simulink model "DriverPath"  (R2025a)
settings: Solver=ode4  StartTime=0.0  StopTime=120  FixedStep=2e-4  RelTol=1e-3
model workspace (MAT data in the model file):
  drvDelayGain = 0.2
  drvKff = 0
  drvKi = 2
  drvKp = 8
  drvN = 4586
  drvNlim = 4
  drvPlanAyCap = 8.6
  drvPlanBrkMargin = 0.6
  drvPlanFW = [-25 -25 -25 -25 -25 -25 -25 -25 -25 -25 -25 -25 ... (4586 elements, 4586x1)]
  drvPlanFzOffN = 0
  drvPlanRH = [10 15 20 25 30 35 40 45 50 55 65 80 ... (39 elements, 13x3)]
  drvPlanRW = [-10 -10 -10 -10 -10 -10 -10 -10 -10 -10 -10 -10 ... (4586 elements, 4586x1)]
  drvPosGainF = 2.5
  drvPosGainR = 2.5
  drvPreviewL = 10
  drvRefKap = [7.37152757629e-05 7.69388209234e-05 7.92839882257e-05 8.08057927362e-05 8.16087590431e-05 8.200862796e-05 8.24299237596e-05 5.11331855999e-05 -0.000149124545088 -0.000317829936074 -0.000343270987749 -0.00029252411928 ... (4586 elements, 4586x1)]
  drvRefPsi = [0 -0.00101392427346 -0.00488065271301 -0.00770746494827 -0.00765908209454 -0.00761399605665 -0.00756111206845 -0.0074887410786 -0.00740766580275 -0.00731954306241 -0.00722036808131 -0.0071279710415 ... (4586 elements, 4586x1)]
  drvRefVplan = [72.4966611223 72.633405974 72.7695456132 72.9050859541 73.0400328206 73.1743919474 73.3081689827 73.4413694893 73.5739989467 73.706062753 73.8375662259 73.968514605 ... (4586 elements, 4586x1)]
  drvRefVraw = [82.8119463936 82.9460939647 83.1011358314 83.2592394893 83.4173431472 83.5753892782 83.7129621785 83.850455756 83.9879220862 84.1191136363 84.2060523792 84.2966104987 ... (4586 elements, 4586x1)]
  drvRefX = [0 0.999999998224 1.99999171552 2.99996181238 3.99993230962 4.99990315023 5.99987433602 6.99984597813 7.99981825196 8.99979110191 9.9997646721 10.999738964 ... (4586 elements, 4586x1)]
  drvRefY = [0 0 -0.00202784084198 -0.0097611965607 -0.0174426181092 -0.0250792109788 -0.0326704630805 -0.0402012910107 -0.0476478052224 -0.0550164870998 -0.0622867605989 -0.0694570977558 ... (4586 elements, 4586x1)]
  drvSFa = 0.9
  drvSFb = 0.9
  drvSpeedLook = 15
  drvTau = 0.05
  drvUsePlan = 1
  drvVScale = 0.95
  drvVnom = 60
  drvVx0 = 82.8119463936
  drvYawGain = 0.2
undefined symbols (not defined in the file): driverTyreGrip, pt, vp
libraries: vehdynlibdriver x1
(part 2 of 2)

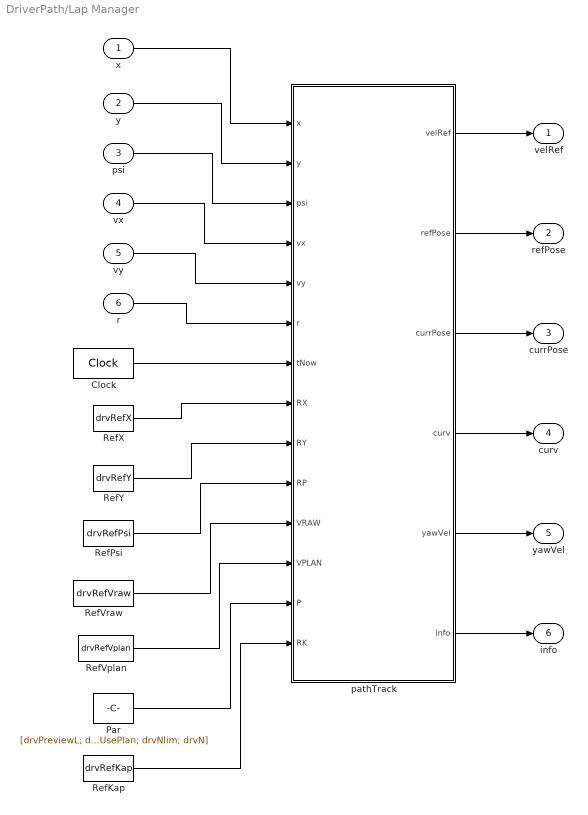
== system DriverPath/Lap Manager ==
  x : Inport
  y : Inport  Port=2
  psi : Inport  Port=3
  vx : Inport  Port=4
  vy : Inport  Port=5
  r : Inport  Port=6
  Clock : DigitalClock  Description=Simulation time, for the lap timer.  SampleTime=0.001
  Par : Constant  Description=Lap Manager parameter vector: [previewL; speedLook; vScale; usePlan; nLim; N]. The last element is the reference-array length drvN -- it was a LITERAL 4586 (Barcelona) until 2026-09-21, which pinned the whole model to one track. drvN is written with drvRefX/Y/Psi/Kap/Vraw/Vplan by simulink/tools/applyTrackPack.m.  Value=[drvPreviewL; drvSpeedLook; drvVScale; drvUsePlan; drvNlim; drvN]
  RefKap : Constant  Description=Racing-line curvature [1/m], ISO sign (+ = LEFT turn), chord-estimated over +-10 m. Feeds the Stanley controller's Curvature port (negated to SAE).  Value=drvRefKap
  RefPsi : Constant  Description=Racing line heading [rad], unwrapped.  Value=drvRefPsi
  RefVplan : Constant  Description=|  Value=drvRefVplan
      | Grip- and feasibility-limited speed profile [m/s]. Built by
      | simulink/tools/buildSpeedPlan.m from the live MF5.2 tyre law, the live
      | ride-height aero and the ECU's own wing-station law; regenerate it with
      | simulink/tools/rebuildDriverPlan.m, which is the supported route and the only
      | TRACKED one (simulink/work/ is git-ignored).
      | 
      | PROVENANCE -- every input is stored beside this vector in the model workspace,
      | and rebuildDriverPlan.m reads AND writes each one, so the plan is exactly
      | reproducible on a fresh clone:
      |   drvPlanRH        measured ride-height-vs-speed table [v RHf RHr]. Must span
      |                    the speeds the car actually reaches -- a table that stops
      |                    short is held at its top row, and held short it once
      |                    predicted ClF = +0.10 at 85-90 m/s where the plant measures
      |                    +0.42, i.e. four times the front LIFT, in the fastest part
      |                    of the lap.
      |   drvPlanAyCap     DRIVER-MODEL lateral ceiling [m/s^2]. The single largest
      |                    lap-time term. It is a limitation of the forward-time
      |                    Stanley + pedal-map driver, NOT a vehicle or aerodynamic
      |                    limit, and must never be quoted as one; raise it when the
      |                    lateral controller improves.
      |   drvPlanFzOffN    residual constant front-axle load transfer [N], ADDITIVE on
      |                    the static load only (never a multiplicative derate of
      |                    static+aero, which would discount front downforce).
      |   drvPlanBrkMargin decel-budget fraction [-].
      |   drvPlanRW/FW     the wing station the ECU's law commands at each point,
      |                    recorded so the plan's aerodynamic assumption is auditable.
      | 
      | The former drvPlanFzF (a multiplicative front derate) is DELETED -- it scaled
      | aerodynamic front load down along with the static load, understating exactly
      | the quantity this project measures.
  RefVraw : Constant  Description=ref.vx(s), the solved ARFWr speed profile [m/s], untouched.  Value=drvRefVraw
  RefX : Constant  Description=Racing line X [m], 1 m uniform, plant start frame.  Value=drvRefX
  RefY : Constant  Description=Racing line Y [m].  Value=drvRefY
  pathTrack : MATLAB Function  TreatAsAtomicUnit=on
  velRef : Outport
  refPose : Outport  Port=2
  currPose : Outport  Port=3
  curv : Outport  Port=4
  yawVel : Outport  Port=5
  info : Outport  Port=6
  wires:
  x/1 -> pathTrack/1(x)
  r/1 -> pathTrack/6(r)
  psi/1 -> pathTrack/3(psi)
  RefVplan/1 -> pathTrack/12(VPLAN)
  y/1 -> pathTrack/2(y)
  vy/1 -> pathTrack/5(vy)
  vx/1 -> pathTrack/4(vx)
  RefX/1 -> pathTrack/8(RX)
  Clock/1 -> pathTrack/7(tNow)
  RefY/1 -> pathTrack/9(RY)
  RefPsi/1 -> pathTrack/10(RP)
  RefVraw/1 -> pathTrack/11(VRAW)
  Par/1 -> pathTrack/13(P)
  RefKap/1 -> pathTrack/14(RK)
  pathTrack/1(velRef) -> velRef/1
  pathTrack/2(refPose) -> refPose/1
  pathTrack/4(curv) -> curv/1
  pathTrack/3(currPose) -> currPose/1
  pathTrack/5(yawVel) -> yawVel/1
  pathTrack/6(info) -> info/1

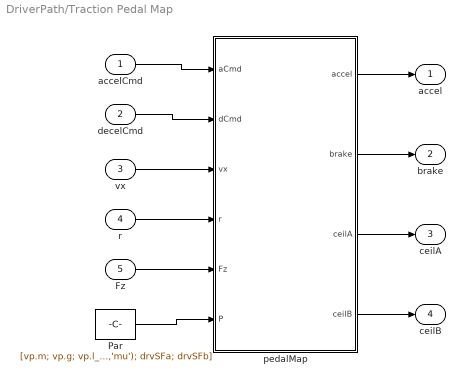
== system DriverPath/Traction Pedal Map ==
  accelCmd : Inport
  decelCmd : Inport  Port=2
  vx : Inport  Port=3
  r : Inport  Port=4
  Fz : Inport  Port=5
  Par : Constant  Description=|  Value=[vp.m; vp.g; vp.l_f; vp.l_r; vp.l; vp.Rw; vp.Tdist; pt.Tmax; vp.gear; pt.Pmax; 1; vp.Tbrake_max; vp.brkB; driverTyreGrip(vp,'mu'); drvSFa; drvSFb]
      | Traction pedal-map parameters, IN THIS ORDER (pedalMap reads them by index):
      |  1 vp.m           mass [kg]
      |  2 vp.g           gravity [m/s^2]
      |  3 vp.l_f         CG -> front axle [m]
      |  4 vp.l_r         CG -> rear axle [m]
      |  5 vp.l           wheelbase [m]
      |  6 vp.Rw          wheel radius [m]
      |  7 vp.Tdist       REAR torque fraction [-]      Parameters/vehParams.m:20
      |  8 pt.Tmax        machine torque cap [Nm]       Parameters/Powertrain.m:80
      |  9 vp.gear        single ratio [-]              Parameters/Powertrain.m:67
      | 10 pt.Pmax        wheel-side power cap [W]      Parameters/Powertrain.m:53
      | 11 Om floor       [rad/s], guards Pmax/Om at standstill -- a numerical guard,
      |                   the one literal in this vector (same role as torqueStep's)
      | 12 vp.Tbrake_max  brake channel cap [Nm]        Parameters/vehParams.m:344
      | 13 vp.brkB        FRONT brake fraction [-]      Parameters/vehParams.m:19
      | 14 muX            PLACEHOLDER tyre peak long. friction (build-time read-back)
      | 15 muY            PLACEHOLDER tyre peak lat. friction  (build-time read-back)
      | 16 drvSFa         accel safety factor [-]  TUNABLE
      | 17 drvSFb         brake safety factor [-]  TUNABLE
  pedalMap : MATLAB Function  TreatAsAtomicUnit=on
  accel : Outport
  brake : Outport  Port=2
  ceilA : Outport  Port=3
  ceilB : Outport  Port=4
  wires:
  accelCmd/1 -> pedalMap/1(aCmd)
  Fz/1 -> pedalMap/5(Fz)
  r/1 -> pedalMap/4(r)
  vx/1 -> pedalMap/3(vx)
  decelCmd/1 -> pedalMap/2(dCmd)
  Par/1 -> pedalMap/6(P)
  pedalMap/1(accel) -> accel/1
  pedalMap/2(brake) -> brake/1
  pedalMap/3(ceilA) -> ceilA/1
  pedalMap/4(ceilB) -> ceilB/1

== matlab function DriverPath/Traction Pedal Map/pedalMap ==
  data: aCmd input; accel output; dCmd input; vx input; r input; Fz input; P input; brake output; ceilA output; ceilB output
function [accel, brake, ceilA, ceilB] = pedalMap(aCmd, dCmd, vx, r, Fz, P)
%#codegen
% Friction-ellipse pedal map. See the subsystem description for the full
% derivation and for WHY this is a multiplicative map and not a clamp.
%
% P = [m; g; l_f; l_r; l; Rw; Tdist; Tmax; gear; Pmax; OmFloor; Tbmax; brkB;
%      muX; muY; SFa; SFb]

mm  = P(1);  lf = P(3);  lr = P(4);  ll = P(5);  Rw = P(6);
Tds = P(7);  Tmx = P(8); gr = P(9);  Pmx = P(10); OmFl = P(11);
Tbm = P(12); brk = P(13); muX = P(14); muY = P(15); SFa = P(16); SFb = P(17);

Fzf = Fz(1) + Fz(2);
Fzr = Fz(3) + Fz(4);

% lateral demand: steady-state ay = vx*r. vx and r are body-integrator
% outputs, so this closes no algebraic loop (VehStateBus.ay would).
ay  = vx*r;
FyF = mm*ay*lr/ll;
FyR = mm*ay*lf/ll;
kxy = muX/muY;

capF = sqrt(max((muX*Fzf)^2 - (kxy*FyF)^2, 0));
capR = sqrt(max((muX*Fzr)^2 - (kxy*FyR)^2, 0));

% drive: same envelope Plant/Torque Path/torqueStep applies
OmM   = max(vx/Rw, OmFl);
TwCap = min(Tmx*gr, Pmx/OmM);
dmdAF = TwCap*(1 - Tds)/Rw;
dmdAR = TwCap*Tds/Rw;
ceilA = min([SFa*capF/max(dmdAF, 1), SFa*capR/max(dmdAR, 1), 1]);

% brake: torqueStep applies T_brake*brkB per FRONT wheel (two wheels)
dmdBF = 2*Tbm*brk/Rw;
dmdBR = 2*Tbm*(1 - brk)/Rw;
ceilB = min([SFb*capF/max(dmdBF, 1), SFb*capR/max(dmdBR, 1), 1]);

ceilA = max(ceilA, 0);
ceilB = max(ceilB, 0);

accel = min(max(aCmd, 0), 1)*ceilA;
brake = min(max(dCmd, 0), 1)*ceilB;

== matlab function DriverPath/Lap Manager/pathTrack ==
  data: x input; velRef output; y input; psi input; vx input; vy input; r input; tNow input; RX input; RY input; RP input; VRAW input; VPLAN input; P input; RK input; refPose output; currPose output; curv output; yawVel output; info output
function [velRef, refPose, currPose, curv, yawVel, info] = pathTrack( ...
        x, y, psi, vx, vy, r, tNow, RX, RY, RP, VRAW, VPLAN, P, RK)
%#codegen
% Path tracker + lap manager.
%
% FRAME: the plant bus, the stored reference and every quantity on LapInfo are
% ISO 8855 (x fwd, y LEFT, psi/r CCW +). The VDB Predictive Driver's Stanley
% controller uses SAE J670 (Z-down): its pose angle is CLOCKWISE positive and
% its hidden coordMode is fixed at "SAE J670 (Z-down)". So the four signals
% handed to the block -- refPose, currPose, curv, yawVel -- are MIRRORED here
% (y, psi, kappa, r all negate; x does not), and the block's SteerCmd is
% mirrored back by the NEGATIVE gain in the Steer scale block. This is the only
% place the driver-side mirror happens, exactly as Plant's Vehicle State Bus
% subsystem is the only place the plant-side mirror happens.
%
% The reference grid is EXACTLY 1 m, closed, so arc length == index - 1.
%
% P = [previewL; speedLook; vScale; usePlan; nLim; N]

Lp   = P(1);  Lv = P(2);  vSc = P(3);  usePlan = P(4);  nLim = P(5);
N    = int32(P(6));

persistent iPrev tStart lapCnt lastLap maxN acquired
if isempty(acquired)
    iPrev = int32(1); tStart = 0; lapCnt = 0; lastLap = 0; maxN = 0;
    acquired = false;
end

% ---- nearest reference point -----------------------------------------
% First step: full search (the car may be started anywhere). After that a
% short forward window is enough -- ds is 1 m and the car covers at most
% 0.12 m per 1 ms step at the reference's peak speed.
best = int32(1); bestD = realmax;
if ~acquired
    for k = 1:N
        dxk = RX(k) - x;  dyk = RY(k) - y;
        dk  = dxk*dxk + dyk*dyk;
        if dk < bestD, bestD = dk; best = int32(k); end
    end
    acquired = true;
else
    for off = -4:40
        k = wrapIdx(iPrev + int32(off), N);
        dxk = RX(k) - x;  dyk = RY(k) - y;
        dk  = dxk*dxk + dyk*dyk;
        if dk < bestD, bestD = dk; best = k; end
    end
end

% ---- lap bookkeeping: detect the index wrapping past the start line ---
if acquired && best < iPrev && (iPrev - best) > (N/2)
    lastLap = tNow - tStart;
    tStart  = tNow;
    lapCnt  = lapCnt + 1;
    maxN    = 0;
end
iPrev = best;

% ---- signed lateral offset from the racing line ----------------------
tx = cos(RP(best));  ty = sin(RP(best));
nOff = tx*(y - RY(best)) - ty*(x - RX(best));   % + = car is LEFT of the line
if abs(nOff) > maxN, maxN = abs(nOff); end

% ---- Stanley reference pose, taken drvPreviewL metres AHEAD of the ----
% nearest point. Stanley's own reference is "the point on the path closest to
% the CG"; a small look-ahead is added because the reference is sampled at 1 m
% and the racing line is not a straight -- it is the same knob the MacAdam
% preview used, so drvPreviewL keeps its meaning.
jp = wrapIdx(best + int32(round(Lp)), N);
dxp = RX(jp) - x;   dyp = RY(jp) - y;
latRef = -sin(psi)*dxp + cos(psi)*dyp;   % logged only, not fed to the block

% MIRROR ISO -> SAE for the block (see the header). ROW vectors: the block's
% RefPose/CurrPose ports are [1x3], and a [3x1] is rejected outright
% (Simulink:Engine:PortDimsMismatch52, measured).
% The reference heading is re-based onto the CAR's heading branch before it is
% handed over. drvRefPsi is UNWRAPPED along the lap (it sweeps -2*pi over one
% lap), so at the start/finish line the stored value jumps by +2*pi while the
% car's psi does not. MEASURED consequence without this: the first lap runs
% clean (max |n| = 1.40 m) and then, the instant the nearest-point index wraps,
% the driver sees a 2*pi heading error and goes to full lock -- 45 deg held, |n|
% growing to 50 m within 7 s. Re-basing makes the handover continuous no matter
% how either signal is wrapped.
ePsi = RP(jp) - psi;
ePsi = ePsi - 2*pi*round(ePsi/(2*pi));
psiRef = psi + ePsi;

refPose  = [RX(jp), -RY(jp), -psiRef];
currPose = [x,      -y,      -psi];
curv     = -RK(jp);

% ---- speed target: the MINIMUM over the look-ahead WINDOW ---------------
% NOT the value at a single point drvSpeedLook metres ahead. Sampling a single
% point ahead has a failure mode that was MEASURED in T2.3: mid-corner, the
% look-ahead point is already past the corner and back on the following faster
% section, so the target RISES and the driver accelerates while still turning.
% Measured at BCN turn 1 with an 80 m single-point look-ahead: the target rose
% 17.5 -> 28.9 m/s through the slow part, the car accelerated 14.3 -> 22.4 m/s
% into a R = 46.5 m corner needing 10.4 m/s^2 of lateral against the placeholder
% tyres' ~8.6, the rear broke away (vy 0.8 -> 18 m/s in 0.7 s) and it spun.
% Taking the MINIMUM over the whole window brakes early AND never asks for speed
% the car has not yet earned; once the slow point is behind, the window holds
% only faster points and the car accelerates out normally.
%
% The loop bound is a compile-time constant with a run-time break, so it is
% codegen-clean and costs at most 401 compares per step.
vT = realmax;
for q = 0:400
    if double(q) > Lv
        break
    end
    jv = wrapIdx(best + int32(q), N);
    if usePlan > 0.5
        vq = VPLAN(jv);
    else
        vq = VRAW(jv);
    end
    if vq < vT
        vT = vq;
    end
end
velRef = vSc*vT;

yawVel = -r;   % SAE

offTrk = 0;
if abs(nOff) > nLim, offTrk = 1; end

info = [double(best) - 1; ...      % 1  sLap [m] (grid is 1 m, 0-based)
        tNow - tStart;    ...      % 2  tLap
        lapCnt;           ...      % 3  lapCount
        lastLap;          ...      % 4  lastLap
        nOff;             ...      % 5  n
        offTrk;           ...      % 6  offTrack
        velRef;           ...      % 7  vTarget
        latRef;           ...      % 8  latRef
        double(best);     ...      % 9  idx
        maxN];            %         10 maxAbsN

function k = wrapIdx(i, N)
%#codegen
k = mod(i - int32(1), N) + int32(1);
